simulink model "sim31"  (R2024a)
settings: Solver=FixedStepAuto  StartTime=0.0  StopTime=10.0  FixedStep=0.25  RelTol=1e-3
settings Model: Creator=alexe  LastModifiedBy=alexe

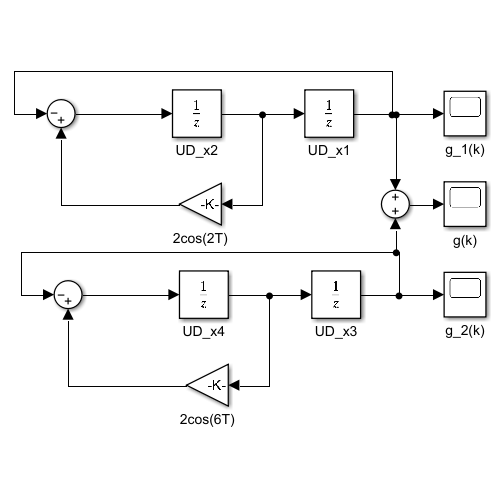
[thumbnail: Simulink's stored preview of the top-level diagram]
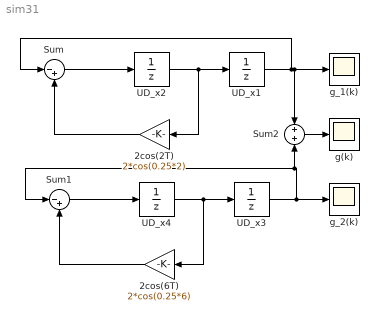
== system sim31 ==
  2cos(2T) : Gain  Gain=2*cos(0.25*2)
  2cos(6T) : Gain  Gain=2*cos(0.25*6)
  Sum : Sum  Inputs=|-+
  Sum1 : Sum  Inputs=|-+
  Sum2 : Sum
  UD_x1 : UnitDelay  SampleTime=-1  HasFrameUpgradeWarning=on
  UD_x2 : UnitDelay  InitialCondition=0.4*sin(0.25*2)  SampleTime=-1  HasFrameUpgradeWarning=on
  UD_x3 : UnitDelay  InitialCondition=2.5  SampleTime=-1  HasFrameUpgradeWarning=on
  UD_x4 : UnitDelay  InitialCondition=2.5*cos(0.25*6)  SampleTime=-1  HasFrameUpgradeWarning=on
  g(k) : Scope
  g_1(k) : Scope
  g_2(k) : Scope
  wires:
  Sum/1 -> UD_x2/1
  2cos(2T)/1 -> Sum/2
  UD_x1/1 -> g_1(k)/1, Sum2/1, Sum/1
  UD_x2/1 -> 2cos(2T)/1, UD_x1/1
  UD_x3/1 -> Sum1/1, Sum2/2, g_2(k)/1
  2cos(6T)/1 -> Sum1/2
  Sum1/1 -> UD_x4/1
  UD_x4/1 -> 2cos(6T)/1, UD_x3/1
  Sum2/1 -> g(k)/1
